simulink model "Robotmodel"  (R2013a)
settings: Solver=ode45  StartTime=0.0  StopTime=run_time  RelTol=1e-3
values from neighbouring files (symbols this model uses):
  cycles = 2    [parameters.m]
  K1 = 4    [parameters.m]
  K2 = 9    [parameters.m]
  K3 = 3    [parameters.m]
  l = .11    (= 0.11)    [parameters.m]
  R = 1    [parameters.m]
  run_time = 251.327    [parameters.m]
libraries: simulink x3
settings Model: Creator=chamanbaz  LastModifiedBy=DevBot

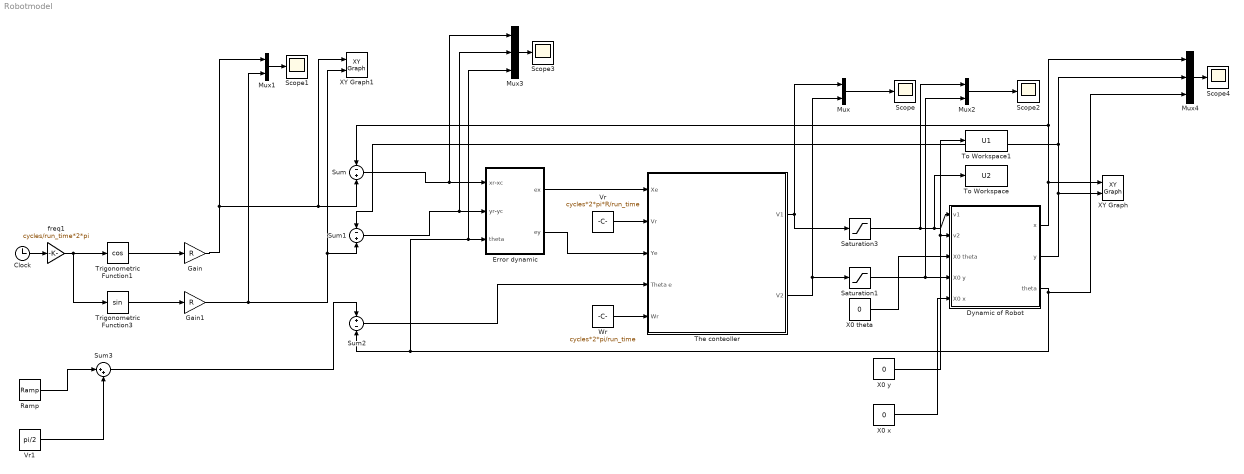
== system Robotmodel ==
  Clock : Clock
  Dynamic of Robot : Subsystem
  Error dynamic : Subsystem
  Gain : Gain  Gain=R
  Gain1 : Gain  Gain=R
  Mux : Mux  Inputs=2
  Mux1 : Mux  Inputs=2
  Mux2 : Mux  Inputs=2
  Mux3 : Mux  Inputs=3
  Mux4 : Mux  Inputs=3
  Ramp : simulink/Sources/Ramp  slope=cycles*2*pi/run_time  start=0  X0=0
  Saturation1 : Saturate  UpperLimit=.15  LowerLimit=-.15
  Saturation3 : Saturate  UpperLimit=.15  LowerLimit=-.15
  Scope{,1..4} (5 alike) : Scope
      Scope1 settings: YMin=0.9  YMax=1.175
      Scope2 settings: SaveName=ScopeData2
      Scope3 settings: YMin=0.9  YMax=1.175  SaveName=ScopeData3
      Scope4 settings: YMin=0.9  YMax=1.175  SaveName=ScopeData4
  Sum : Sum  Inputs=-|+
  Sum1 : Sum  Inputs=-|+
  Sum2 : Sum  Inputs=+|-
  Sum3 : Sum  Inputs=|++
  The conteoller : Subsystem
  To Workspace : ToWorkspace  VariableName=U2  SampleTime=0.3  SaveFormat=Timeseries
  To Workspace1 : ToWorkspace  VariableName=U1  SampleTime=0.3  SaveFormat=Timeseries
  Trigonometric Function1 : Trigonometry  Operator=cos
  Trigonometric Function3 : Trigonometry
  Vr : Constant  Value=cycles*2*pi*R/run_time
  Vr1 : Constant  Value=pi/2
  Wr : Constant  Value=cycles*2*pi/run_time
  X0 theta : Constant  Value=0
  X0 x : Constant  Value=0
  X0 y : Constant  Value=0
  XY Graph : simulink/Sinks/XY Graph  xmin=-1  xmax=1  ymin=-1  ymax=1.5  st=-1
  XY Graph1 : simulink/Sinks/XY Graph  xmin=-2  xmax=2  ymin=-2  ymax=2  st=-1
  freq1 : Gain  Gain=cycles/run_time*2*pi
  wires:
  Gain/1 -> Mux1/1, XY Graph1/1, Sum/2
  Gain1/1 -> Mux1/2, XY Graph1/2, Sum1/2
  Error dynamic/1(ex) -> The conteoller/1(Xe)
  Error dynamic/2(ey) -> The conteoller/3(Ye)
  Sum2/1 -> The conteoller/4(Theta e)
  Sum/1 -> Mux3/1, Error dynamic/1(xr-xc)
  Sum1/1 -> Mux3/2, Error dynamic/2(yr-yc)
  Clock/1 -> freq1/1
  Trigonometric Function1/1 -> Gain/1
  Trigonometric Function3/1 -> Gain1/1
  freq1/1 -> Trigonometric Function1/1, Trigonometric Function3/1
  Ramp/1 -> Sum3/1
  Vr1/1 -> Sum3/2
  Sum3/1 -> Sum2/1
  Vr/1 -> The conteoller/2(Vr)
  Wr/1 -> The conteoller/5(Wr)
  Mux/1 -> Scope/1
  Mux1/1 -> Scope1/1
  Mux2/1 -> Scope2/1
  The conteoller/1(V1) -> Saturation3/1, Mux/1
  X0 theta/1 -> Dynamic of Robot/3(X0 theta)
  X0 y/1 -> Dynamic of Robot/4(X0 y)
  X0 x/1 -> Dynamic of Robot/5(X0 x)
  Mux3/1 -> Scope3/1
  Dynamic of Robot/3(theta) -> Mux4/3, Mux3/3, Error dynamic/3(theta), Sum2/2
  Dynamic of Robot/1(x) -> XY Graph/1, Mux4/1, Sum/1
  Dynamic of Robot/2(y) -> Mux4/2, Sum1/1, XY Graph/2
  Mux4/1 -> Scope4/1
  The conteoller/2(V2) -> Saturation1/1, Mux/2
  Saturation3/1 -> Mux2/1, To Workspace/1, Dynamic of Robot/1(v1)
  Saturation1/1 -> Mux2/2, To Workspace1/1, Dynamic of Robot/2(v2)

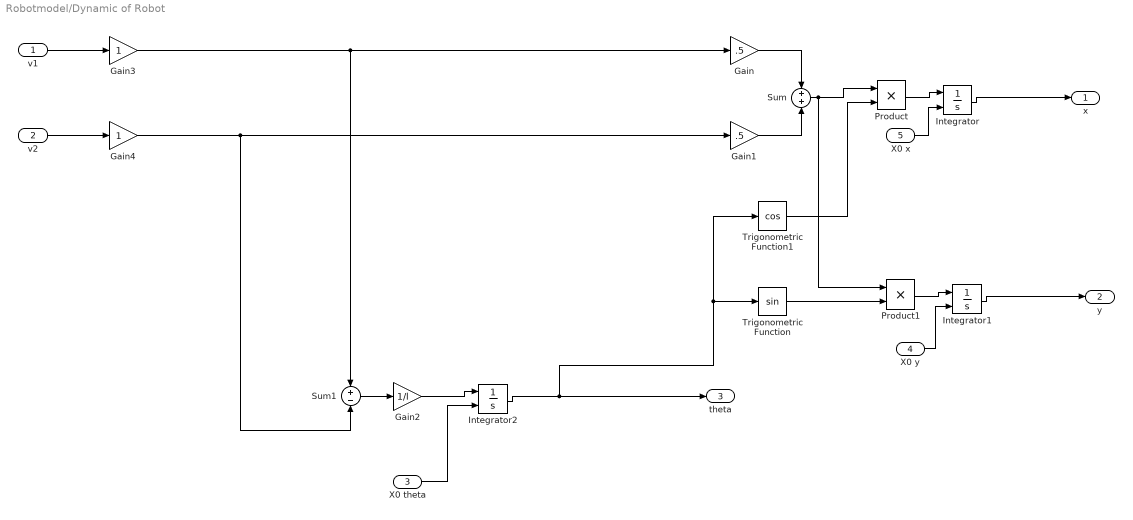
== system Robotmodel/Dynamic of Robot ==
  v1 : Inport
  v2 : Inport  Port=2
  X0 theta : Inport  Port=3
  X0 y : Inport  Port=4
  X0 x : Inport  Port=5
  Gain : Gain  Gain=.5
  Gain1 : Gain  Gain=.5
  Gain2 : Gain  Gain=1/l
  Gain3 : Gain
  Gain4 : Gain
  Integrator : Integrator  InitialConditionSource=external
  Integrator1 : Integrator  InitialConditionSource=external
  Integrator2 : Integrator  InitialConditionSource=external  InitialCondition=pi
  Product : Product
  Product1 : Product
  Sum : Sum  Inputs=+|+
  Sum1 : Sum  Inputs=+|-
  Trigonometric Function : Trigonometry
  Trigonometric Function1 : Trigonometry  Operator=cos
  x : Outport
  y : Outport  Port=2
  theta : Outport  Port=3
  wires:
  Integrator1/1 -> y/1
  Integrator/1 -> x/1
  Gain/1 -> Sum/1
  Gain1/1 -> Sum/2
  Product/1 -> Integrator/1
  Sum/1 -> Product1/1, Product/1
  Trigonometric Function1/1 -> Product/2
  Trigonometric Function/1 -> Product1/2
  Product1/1 -> Integrator1/1
  v2/1 -> Gain4/1
  v1/1 -> Gain3/1
  Gain2/1 -> Integrator2/1
  Sum1/1 -> Gain2/1
  Integrator2/1 -> theta/1, Trigonometric Function1/1, Trigonometric Function/1
  X0 theta/1 -> Integrator2/2
  X0 y/1 -> Integrator1/2
  X0 x/1 -> Integrator/2
  Gain3/1 -> Sum1/1, Gain/1
  Gain4/1 -> Sum1/2, Gain1/1

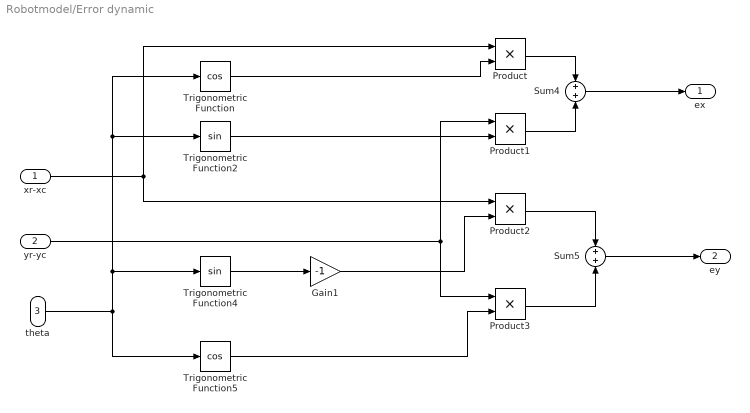
== system Robotmodel/Error dynamic ==
  xr-xc : Inport
  yr-yc : Inport  Port=2
  theta : Inport  Port=3
  Gain1 : Gain  Gain=-1
  Product{,1..3} (4 alike) : Product
  Sum4 : Sum  Inputs=+|+
  Sum5 : Sum  Inputs=+|+
  Trigonometric Function : Trigonometry  Operator=cos
  Trigonometric Function2 : Trigonometry
  Trigonometric Function4 : Trigonometry
  Trigonometric Function5 : Trigonometry  Operator=cos
  ex : Outport
  ey : Outport  Port=2
  wires:
  Trigonometric Function2/1 -> Product1/2
  Sum5/1 -> ey/1
  Sum4/1 -> ex/1
  Trigonometric Function/1 -> Product/2
  Product1/1 -> Sum4/2
  Product3/1 -> Sum5/2
  theta/1 -> Trigonometric Function5/1, Trigonometric Function4/1, Trigonometric Function2/1, Trigonometric Function/1
  xr-xc/1 -> Product/1, Product2/1
  Product/1 -> Sum4/1
  Trigonometric Function5/1 -> Product3/2
  Trigonometric Function4/1 -> Gain1/1
  yr-yc/1 -> Product1/1, Product3/1
  Gain1/1 -> Product2/2
  Product2/1 -> Sum5/1

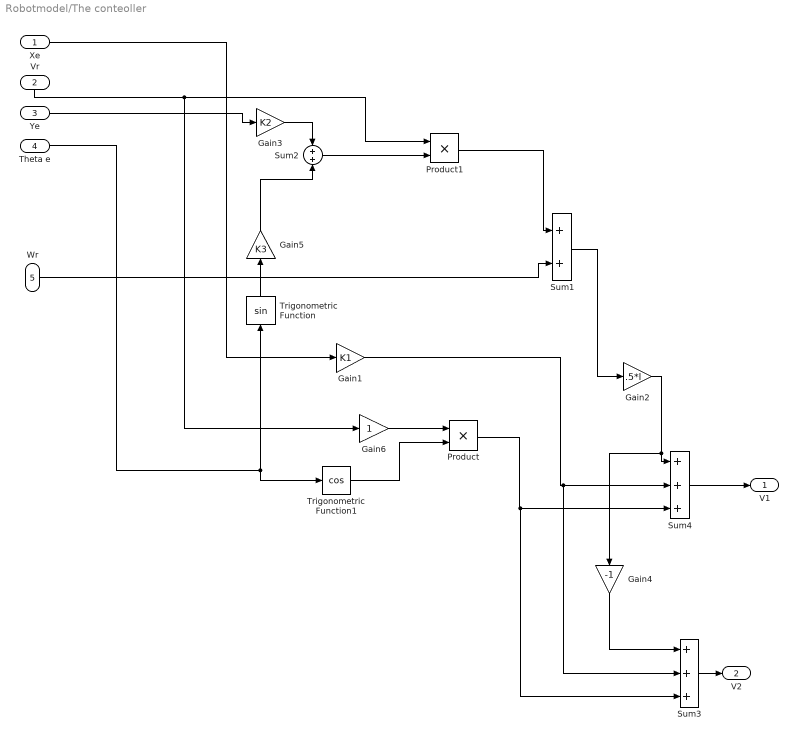
== system Robotmodel/The conteoller ==
  Xe : Inport
  Vr : Inport  Port=2
  Ye : Inport  Port=3
  Theta e : Inport  Port=4
  Wr : Inport  Port=5
  Gain1 : Gain  Gain=K1
  Gain2 : Gain  Gain=.5*l
  Gain3 : Gain  Gain=K2
  Gain4 : Gain  Gain=-1
  Gain5 : Gain  Gain=K3
  Gain6 : Gain
  Product : Product
  Product1 : Product
  Sum1 : Sum
  Sum2 : Sum
  Sum3 : Sum  Inputs=+++
  Sum4 : Sum  Inputs=+++
  Trigonometric Function : Trigonometry
  Trigonometric Function1 : Trigonometry  Operator=cos
  V1 : Outport
  V2 : Outport  Port=2
  wires:
  Product/1 -> Sum3/3, Sum4/3
  Xe/1 -> Gain1/1
  Gain1/1 -> Sum3/2, Sum4/2
  Gain2/1 -> Gain4/1, Sum4/1
  Theta e/1 -> Trigonometric Function1/1, Trigonometric Function/1
  Vr/1 -> Gain6/1, Product1/1
  Trigonometric Function1/1 -> Product/2
  Wr/1 -> Sum1/2
  Product1/1 -> Sum1/1
  Ye/1 -> Gain3/1
  Gain3/1 -> Sum2/1
  Trigonometric Function/1 -> Gain5/1
  Sum2/1 -> Product1/2
  Sum1/1 -> Gain2/1
  Gain4/1 -> Sum3/1
  Sum3/1 -> V2/1
  Gain5/1 -> Sum2/2
  Sum4/1 -> V1/1
  Gain6/1 -> Product/1
